simulink model "Observador"  (R2023b)
settings: Solver=VariableStepAuto  StartTime=0.0  StopTime=10.0  RelTol=1e-3
values from neighbouring files (symbols this model uses):
  J_nom = 1.9785e-5    (= 1.9785e-05)    [Controlador.m]    (also in varLC.m = 1.97847222222e-05)
  K_obs_theta = 6400    [Controlador.m]    (also in varLC.m)
  K_obs_w = 10240000    [Controlador.m]    (also in varLC.m)
settings Model: Creator=gonza  LastModifiedBy=tomas

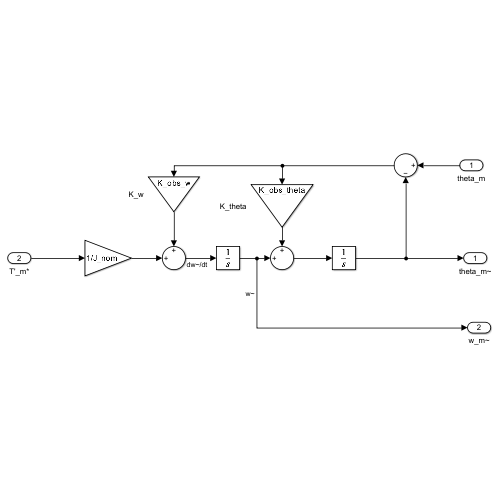
[thumbnail: Simulink's stored preview of the top-level diagram]
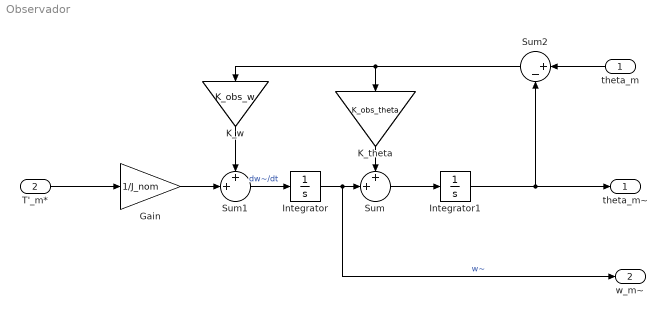
== system Observador ==
  theta_m : Inport
  T'_m* : Inport  Port=2
  Gain : Gain  Gain=1/J_nom
  Integrator : Integrator
  Integrator1 : Integrator
  K_theta : Gain  Gain=K_obs_theta
  K_w : Gain  Gain=K_obs_w
  Sum : Sum  Inputs=++|
  Sum1 : Sum  Inputs=++|
  Sum2 : Sum  Inputs=|+-
  theta_m~ : Outport
  w_m~ : Outport  Port=2
  wires:
  T'_m*/1 -> Gain/1
  Integrator1/1 -> theta_m~/1, Sum2/2
  theta_m/1 -> Sum2/1
  K_theta/1 -> Sum/1
  K_w/1 -> Sum1/1
  Sum2/1 -> K_w/1, K_theta/1
  Gain/1 -> Sum1/2
  Sum1/1 -> Integrator/1  "dw~/dt"
  Integrator/1 -> w_m~/1, Sum/2  "w~"
  Sum/1 -> Integrator1/1
